simulink model "Sistemi_Lineari"  (R2020b)
settings: Solver=VariableStepAuto  StartTime=0.0  StopTime=30  MaxStep=0.1  RelTol=1e-3
undefined symbols (not defined in the file or in its folder): D, K, M
libraries: cstblocks x1
settings Model: Creator=Stefano  LastModifiedBy=Stefano

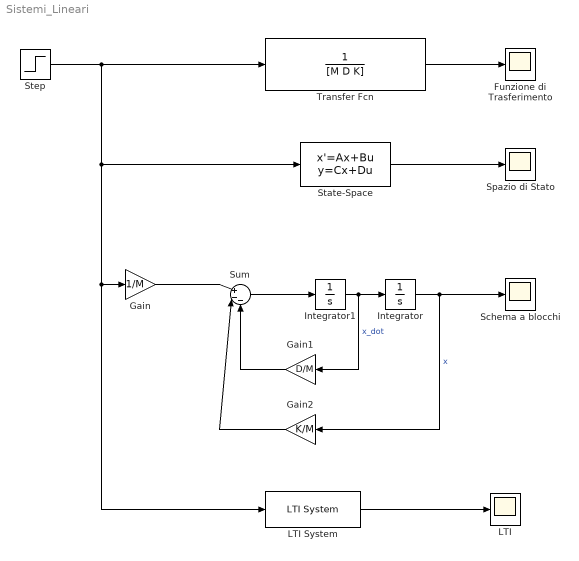
== system Sistemi_Lineari ==
  Funzione di Trasferimento : Scope
  Gain : Gain  Gain=1/M
  Gain1 : Gain  Gain=D/M
  Gain2 : Gain  Gain=K/M
  Integrator : Integrator
  Integrator1 : Integrator
  LTI : Scope
  LTI System : cstblocks/LTI System  sys=F  IC=[]
  Schema a blocchi : Scope
  Spazio di Stato : Scope
  State-Space : StateSpace  A=[0 1 ; -K/M -D/M]  B=[0 ; 1/M]  C=[1 0]  D=0  InitialCondition=0
  Step : Step  SampleTime=0
  Sum : Sum  Inputs=|+--
  Transfer Fcn : TransferFcn  Denominator=[M D K]
  wires:
  Step/1 -> Transfer Fcn/1, LTI System/1, Gain/1, State-Space/1
  Transfer Fcn/1 -> Funzione di Trasferimento/1
  State-Space/1 -> Spazio di Stato/1
  Integrator1/1 -> Gain1/1, Integrator/1  "x_dot"
  Integrator/1 -> Schema a blocchi/1, Gain2/1  "x"
  Sum/1 -> Integrator1/1
  Gain1/1 -> Sum/3
  Gain2/1 -> Sum/2
  Gain/1 -> Sum/1
  LTI System/1 -> LTI/1
